simulink library "PD_Controller_Lib_old"  (R2018b)
settings: Solver=VariableStepAuto  StartTime=0.0  StopTime=10.0  RelTol=1e-3
undefined symbols (not defined in the file): fswParams
libraries: aerolibutil x2
settings Model: Creator=devantormey  LastModifiedBy=colem

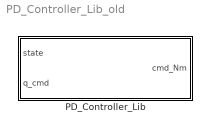
== system PD_Controller_Lib_old ==
  PD_Controller_Lib : Subsystem

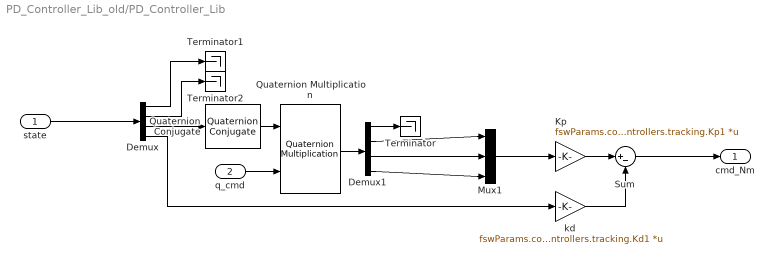
== system PD_Controller_Lib_old/PD_Controller_Lib ==
  state : Inport
  q_cmd : Inport  Port=2
  Demux : Demux  Outputs=[3 3 4 3]
  Demux1 : Demux
  Kp : Gain  Gain=fswParams.controllers.tracking.Kp1  Multiplication=Matrix(K*u)
  Mux1 : Mux  Inputs=3
  Quaternion Conjugate : aerolibutil/Quaternion Conjugate
      settings: SourceProductName=Aerospace Blockset  SourceProductBaseCode=AE
  Quaternion Multiplication : aerolibutil/Quaternion Multiplication
  Sum : Sum  Inputs=|+-
  Terminator : Terminator
  Terminator1 : Terminator
  Terminator2 : Terminator
  kd : Gain  Gain=fswParams.controllers.tracking.Kd1  Multiplication=Matrix(K*u)
  cmd_Nm : Outport
  wires:
  Demux1/3 -> Mux1/2
  Kp/1 -> Sum/1
  Demux1/4 -> Mux1/3
  Mux1/1 -> Kp/1
  Demux1/2 -> Mux1/1
  q_cmd/1 -> Quaternion Multiplication/2
  Quaternion Conjugate/1 -> Quaternion Multiplication/1
  kd/1 -> Sum/2
  Quaternion Multiplication/1 -> Demux1/1
  Demux1/1 -> Terminator/1
  Demux/3 -> Quaternion Conjugate/1
  Demux/4 -> kd/1
  Demux/1 -> Terminator1/1
  Demux/2 -> Terminator2/1
  state/1 -> Demux/1
  Sum/1 -> cmd_Nm/1
